simulink library "inp"  (R2021b)
settings: Solver=VariableStepAuto  StartTime=0.0  StopTime=10.0  RelTol=1e-3
undefined symbols (not defined in the file): C_TASK_5MS_S, FALSE, KINP_AcoreReadyToSlp_flg_ovrdflg, KINP_AcoreReadyToSlp_flg_ovrdval, KINP_AllowMovThd_OTA_enum_ovrdflg, KINP_AllowMovThd_OTA_enum_ovrdval, KINP_APSAngleTarget_Deg_ovrdflg, KINP_APSAngleTarget_Deg_ovrdval, KINP_APSDecReq_mps2_ovrdflg, KINP_APSDecReq_mps2_ovrdval, KINP_APSDecReqA_flg_ovrdflg, KINP_APSDecReqA_flg_ovrdval, KINP_APSDFLL_cm_ovrdflg, KINP_APSDFLL_cm_ovrdval, KINP_APSDFLR_cm_ovrdflg, KINP_APSDFLR_cm_ovrdval, KINP_APSDRLL_cm_ovrdflg, KINP_APSDRLL_cm_ovrdval, KINP_APSDRLR_cm_ovrdflg, KINP_APSDRLR_cm_ovrdval, KINP_APSExitCondition_enum_ovrdflg, KINP_APSExitCondition_enum_ovrdval, KINP_APSHWVer_enum_ovrdflg, KINP_APSHWVer_enum_ovrdval, KINP_APSProgressPCT_pct_ovrdflg, KINP_APSProgressPCT_pct_ovrdval, KINP_APSPwrReq_enum_ovrdflg, KINP_APSPwrReq_enum_ovrdval, KINP_APSReq_enum_ovrdflg, KINP_APSReq_enum_ovrdval, KINP_APSRQDisplay_enum_ovrdflg, KINP_APSRQDisplay_enum_ovrdval, KINP_APSRqEPASCtrl_flg_ovrdflg, KINP_APSRqEPASCtrl_flg_ovrdval, KINP_APSShiftPosnReq_enum_ovrdval, KINP_APSShiftPosnReq_enum_ovrflg, KINP_APSSpeedCMD_kph_ovrdval, KINP_APSSpeedCMD_kph_ovrflg, KINP_APSStaSystem_enum_ovrdflg, KINP_APSStaSystem_enum_ovrdval, KINP_APSSWVer_enum_ovrdflg, KINP_APSSWVer_enum_ovrdval, KINP_APSVMCReqA_flg_ovrdval, KINP_APSVMCReqA_flg_ovrflg, KINP_APSVRqEPASCtrl_flg_ovrdflg, KINP_APSVRqEPASCtrl_flg_ovrdval, KINP_AuxBattVolmV_mV_ovrdflg, KINP_AuxBattVolmV_mV_ovrdval, KINP_CAASSta_enum_ovrdflg, KINP_CAASSta_enum_ovrdval, KINP_CAASVMCReqA_flg_ovrdval, KINP_CAASVMCReqA_flg_ovrflg, KINP_CAN1BusOff_flg_ovrdflg, KINP_CAN1BusOff_flg_ovrdval, KINP_CAN2BusOff_flg_ovrdflg, KINP_CAN2BusOff_flg_ovrdval, KINP_CAN3BusOff_flg_ovrdflg, KINP_CAN3BusOff_flg_ovrdval, KINP_CAN4BusOff_flg_ovrdflg, KINP_CAN4BusOff_flg_ovrdval ... (+152)
libraries: FVT_lib x1037, hcu_lib x1
(part 31 of 34)

== system inp/INP/CAN4/SignalCheck/zGW_LINDr2 ==
  BHAL_outputs : Inport
  inp_CanValid_bus : Inport  Port=2
  ACT1ResponseError : FVT_lib/inp/can_signal_template  SystemSampleTime=-1  VariantActivationTime=update diagram  Latency=0  AutoFrameSizeCalculation=off
      link override defval: Value=KINP_ACT1ResponseError_flg_defval
      link override ovrdflg: Value=KINP_ACT1ResponseError_flg_ovrdflg
      link override ovrdval: Value=KINP_ACT1ResponseError_flg_ovrdval
  Terminator_1 : Terminator
  True_VHAL_ACT1ResponseError_flg : Constant  Value=TRUE  OutDataTypeStr=boolean
  slr1_1 : BusSelector  OutputSignals=VINP_CANMsgValidzGWLINDr2_flg
  slr_VHAL_ACT1ResponseError_flg : BusSelector  OutputSignals=VHAL_ACT1ResponseError_flg
  VINP_ACT1ResponseError_flg : Outport
  wires:
  BHAL_outputs/1 -> [BHAL_outputs]
  inp_CanValid_bus/1 -> [inp_CanValid_bus]
  [BHAL_outputs] -> slr_VHAL_ACT1ResponseError_flg/1
  slr_VHAL_ACT1ResponseError_flg/1 -> ACT1ResponseError/1  "<VHAL_ACT1ResponseError_flg>"
  True_VHAL_ACT1ResponseError_flg/1 -> ACT1ResponseError/2
  [inp_CanValid_bus] -> slr1_1/1
  slr1_1/1 -> ACT1ResponseError/3  "<VINP_CANMsgValidzGWLINDr2_flg>"
  ACT1ResponseError/1 -> VINP_ACT1ResponseError_flg/1  "VINP_ACT1ResponseError_flg"
  ACT1ResponseError/2 -> Terminator_1/1

== system inp/INP/CAN4/SignalCheck/zGW_LINFr1 ==
  BHAL_outputs : Inport
  inp_CanValid_bus : Inport  Port=2
  AGSActualPosition : FVT_lib/inp/can_signal_template  SystemSampleTime=-1  VariantActivationTime=update diagram  Latency=0  AutoFrameSizeCalculation=off
      link override defval: Value=KINP_AGSActualPosition_enum_defval
      link override ovrdflg: Value=KINP_AGSActualPosition_enum_ovrdflg
      link override ovrdval: Value=KINP_AGSActualPosition_enum_ovrdval
  FGSIntenRspSta : FVT_lib/inp/can_signal_template  SystemSampleTime=-1  VariantActivationTime=update diagram  Latency=0  AutoFrameSizeCalculation=off
      link override defval: Value=KINP_FGSIntenRspSta_enum_defval
      link override ovrdflg: Value=KINP_FGSIntenRspSta_enum_ovrdflg
      link override ovrdval: Value=KINP_FGSIntenRspSta_enum_ovrdval
  Terminator_1 : Terminator
  Terminator_2 : Terminator
  True_VHAL_AGSActualPosition_enum : Constant  Value=TRUE  OutDataTypeStr=boolean
  True_VHAL_FGSIntenRspSta_enum : Constant  Value=TRUE  OutDataTypeStr=boolean
  slr1_1 : BusSelector  OutputSignals=VINP_CANMsgValidzGWLINFr1_flg
  slr1_2 : BusSelector  OutputSignals=VINP_CANMsgValidzGWLINFr1_flg
  slr_VHAL_AGSActualPosition_enum : BusSelector  OutputSignals=VHAL_AGSActualPosition_enum
  slr_VHAL_FGSIntenRspSta_enum : BusSelector  OutputSignals=VHAL_FGSIntenRspSta_enum
  VINP_AGSActualPosition_enum : Outport
  VINP_FGSIntenRspSta_enum : Outport  Port=2
  wires:
  BHAL_outputs/1 -> [BHAL_outputs]
  inp_CanValid_bus/1 -> [inp_CanValid_bus]
  [BHAL_outputs] -> slr_VHAL_AGSActualPosition_enum/1
  slr_VHAL_AGSActualPosition_enum/1 -> AGSActualPosition/1  "<VHAL_AGSActualPosition_enum>"
  True_VHAL_AGSActualPosition_enum/1 -> AGSActualPosition/2
  [inp_CanValid_bus] -> slr1_1/1
  slr1_1/1 -> AGSActualPosition/3  "<VINP_CANMsgValidzGWLINFr1_flg>"
  AGSActualPosition/1 -> VINP_AGSActualPosition_enum/1  "VINP_AGSActualPosition_enum"
  AGSActualPosition/2 -> Terminator_1/1
  [BHAL_outputs] -> slr_VHAL_FGSIntenRspSta_enum/1
  slr_VHAL_FGSIntenRspSta_enum/1 -> FGSIntenRspSta/1  "<VHAL_FGSIntenRspSta_enum>"
  True_VHAL_FGSIntenRspSta_enum/1 -> FGSIntenRspSta/2
  [inp_CanValid_bus] -> slr1_2/1
  slr1_2/1 -> FGSIntenRspSta/3  "<VINP_CANMsgValidzGWLINFr1_flg>"
  FGSIntenRspSta/1 -> VINP_FGSIntenRspSta_enum/1  "VINP_FGSIntenRspSta_enum"
  FGSIntenRspSta/2 -> Terminator_2/1

== system inp/INP/CAN4/SignalCheck/zGW_LINFr2 ==
  BHAL_outputs : Inport
  inp_CanValid_bus : Inport  Port=2
  EWP1BlockError : FVT_lib/inp/can_signal_template  SystemSampleTime=-1  VariantActivationTime=update diagram  Latency=0  AutoFrameSizeCalculation=off
      link override defval: Value=KINP_EWP1BlockError_enum_defval
      link override ovrdflg: Value=KINP_EWP1BlockError_enum_ovrdflg
      link override ovrdval: Value=KINP_EWP1BlockError_enum_ovrdval
  EWP1OverCurrError : FVT_lib/inp/can_signal_template  SystemSampleTime=-1  VariantActivationTime=update diagram  Latency=0  AutoFrameSizeCalculation=off
      link override defval: Value=KINP_EWP1OverCurrError_enum_defval
      link override ovrdflg: Value=KINP_EWP1OverCurrError_enum_ovrdflg
      link override ovrdval: Value=KINP_EWP1OverCurrError_enum_ovrdval
  EWP2BlockError : FVT_lib/inp/can_signal_template  SystemSampleTime=-1  VariantActivationTime=update diagram  Latency=0  AutoFrameSizeCalculation=off
      link override defval: Value=KINP_EWP2BlockError_enum_defval
      link override ovrdflg: Value=KINP_EWP2BlockError_enum_ovrdflg
      link override ovrdval: Value=KINP_EWP2BlockError_enum_ovrdval
  EWP2OverCurrError : FVT_lib/inp/can_signal_template  SystemSampleTime=-1  VariantActivationTime=update diagram  Latency=0  AutoFrameSizeCalculation=off
      link override defval: Value=KINP_EWP2OverCurrError_enum_defval
      link override ovrdflg: Value=KINP_EWP2OverCurrError_enum_ovrdflg
      link override ovrdval: Value=KINP_EWP2OverCurrError_enum_ovrdval
  EWP3BlockError : FVT_lib/inp/can_signal_template  SystemSampleTime=-1  VariantActivationTime=update diagram  Latency=0  AutoFrameSizeCalculation=off
      link override defval: Value=KINP_EWP3BlockError_enum_defval
      link override ovrdflg: Value=KINP_EWP3BlockError_enum_ovrdflg
      link override ovrdval: Value=KINP_EWP3BlockError_enum_ovrdval
  EWP3OverCurrError : FVT_lib/inp/can_signal_template  SystemSampleTime=-1  VariantActivationTime=update diagram  Latency=0  AutoFrameSizeCalculation=off
      link override defval: Value=KINP_EWP3OverCurrError_enum_defval
      link override ovrdflg: Value=KINP_EWP3OverCurrError_enum_ovrdflg
      link override ovrdval: Value=KINP_EWP3OverCurrError_enum_ovrdval
  Terminator_{1..6} (6 alike) : Terminator
  True_VHAL_EWP1BlockError_enum : Constant  Value=TRUE  OutDataTypeStr=boolean
  True_VHAL_EWP1OverCurrError_enum : Constant  Value=TRUE  OutDataTypeStr=boolean
  True_VHAL_EWP2BlockError_enum : Constant  Value=TRUE  OutDataTypeStr=boolean
  True_VHAL_EWP2OverCurrError_enum : Constant  Value=TRUE  OutDataTypeStr=boolean
  True_VHAL_EWP3BlockError_enum : Constant  Value=TRUE  OutDataTypeStr=boolean
  True_VHAL_EWP3OverCurrError_enum : Constant  Value=TRUE  OutDataTypeStr=boolean
  slr1_{1..6} (6 alike) : BusSelector  OutputSignals=VINP_CANMsgValidzGWLINFr2_flg
  slr_VHAL_EWP1BlockError_enum : BusSelector  OutputSignals=VHAL_EWP1BlockError_enum
  slr_VHAL_EWP1OverCurrError_enum : BusSelector  OutputSignals=VHAL_EWP1OverCurrError_enum
  slr_VHAL_EWP2BlockError_enum : BusSelector  OutputSignals=VHAL_EWP2BlockError_enum
  slr_VHAL_EWP2OverCurrError_enum : BusSelector  OutputSignals=VHAL_EWP2OverCurrError_enum
  slr_VHAL_EWP3BlockError_enum : BusSelector  OutputSignals=VHAL_EWP3BlockError_enum
  slr_VHAL_EWP3OverCurrError_enum : BusSelector  OutputSignals=VHAL_EWP3OverCurrError_enum
  VINP_EWP1BlockError_enum : Outport
  VINP_EWP1OverCurrError_enum : Outport  Port=2
  VINP_EWP2BlockError_enum : Outport  Port=3
  VINP_EWP2OverCurrError_enum : Outport  Port=4
  VINP_EWP3BlockError_enum : Outport  Port=5
  VINP_EWP3OverCurrError_enum : Outport  Port=6
  wires:
  BHAL_outputs/1 -> [BHAL_outputs]
  inp_CanValid_bus/1 -> [inp_CanValid_bus]
  [BHAL_outputs] -> slr_VHAL_EWP1BlockError_enum/1
  slr_VHAL_EWP1BlockError_enum/1 -> EWP1BlockError/1  "<VHAL_EWP1BlockError_enum>"
  True_VHAL_EWP1BlockError_enum/1 -> EWP1BlockError/2
  [inp_CanValid_bus] -> slr1_1/1
  slr1_1/1 -> EWP1BlockError/3  "<VINP_CANMsgValidzGWLINFr2_flg>"
  EWP1BlockError/1 -> VINP_EWP1BlockError_enum/1  "VINP_EWP1BlockError_enum"
  EWP1BlockError/2 -> Terminator_1/1
  [BHAL_outputs] -> slr_VHAL_EWP1OverCurrError_enum/1
  slr_VHAL_EWP1OverCurrError_enum/1 -> EWP1OverCurrError/1  "<VHAL_EWP1OverCurrError_enum>"
  True_VHAL_EWP1OverCurrError_enum/1 -> EWP1OverCurrError/2
  [inp_CanValid_bus] -> slr1_2/1
  slr1_2/1 -> EWP1OverCurrError/3  "<VINP_CANMsgValidzGWLINFr2_flg>"
  EWP1OverCurrError/1 -> VINP_EWP1OverCurrError_enum/1  "VINP_EWP1OverCurrError_enum"
  EWP1OverCurrError/2 -> Terminator_2/1
  [BHAL_outputs] -> slr_VHAL_EWP2BlockError_enum/1
  slr_VHAL_EWP2BlockError_enum/1 -> EWP2BlockError/1  "<VHAL_EWP2BlockError_enum>"
  True_VHAL_EWP2BlockError_enum/1 -> EWP2BlockError/2
  [inp_CanValid_bus] -> slr1_3/1
  slr1_3/1 -> EWP2BlockError/3  "<VINP_CANMsgValidzGWLINFr2_flg>"
  EWP2BlockError/1 -> VINP_EWP2BlockError_enum/1  "VINP_EWP2BlockError_enum"
  EWP2BlockError/2 -> Terminator_3/1
  [BHAL_outputs] -> slr_VHAL_EWP2OverCurrError_enum/1
  slr_VHAL_EWP2OverCurrError_enum/1 -> EWP2OverCurrError/1  "<VHAL_EWP2OverCurrError_enum>"
  True_VHAL_EWP2OverCurrError_enum/1 -> EWP2OverCurrError/2
  [inp_CanValid_bus] -> slr1_4/1
  slr1_4/1 -> EWP2OverCurrError/3  "<VINP_CANMsgValidzGWLINFr2_flg>"
  EWP2OverCurrError/1 -> VINP_EWP2OverCurrError_enum/1  "VINP_EWP2OverCurrError_enum"
  EWP2OverCurrError/2 -> Terminator_4/1
  [BHAL_outputs] -> slr_VHAL_EWP3BlockError_enum/1
  slr_VHAL_EWP3BlockError_enum/1 -> EWP3BlockError/1  "<VHAL_EWP3BlockError_enum>"
  True_VHAL_EWP3BlockError_enum/1 -> EWP3BlockError/2
  [inp_CanValid_bus] -> slr1_5/1
  slr1_5/1 -> EWP3BlockError/3  "<VINP_CANMsgValidzGWLINFr2_flg>"
  EWP3BlockError/1 -> VINP_EWP3BlockError_enum/1  "VINP_EWP3BlockError_enum"
  EWP3BlockError/2 -> Terminator_5/1
  [BHAL_outputs] -> slr_VHAL_EWP3OverCurrError_enum/1
  slr_VHAL_EWP3OverCurrError_enum/1 -> EWP3OverCurrError/1  "<VHAL_EWP3OverCurrError_enum>"
  True_VHAL_EWP3OverCurrError_enum/1 -> EWP3OverCurrError/2
  [inp_CanValid_bus] -> slr1_6/1
  slr1_6/1 -> EWP3OverCurrError/3  "<VINP_CANMsgValidzGWLINFr2_flg>"
  EWP3OverCurrError/1 -> VINP_EWP3OverCurrError_enum/1  "VINP_EWP3OverCurrError_enum"
  EWP3OverCurrError/2 -> Terminator_6/1

== system inp/INP/CAN4/SignalCheck/zGW_SEAT1 ==
  BHAL_outputs : Inport
  inp_CanValid_bus : Inport  Port=2
  DSEATAntiSta : FVT_lib/inp/can_signal_template  SystemSampleTime=-1  VariantActivationTime=update diagram  Latency=0  AutoFrameSizeCalculation=off
      link override defval: Value=KINP_DSEATAntiSta_flg_defval
      link override ovrdflg: Value=KINP_DSEATAntiSta_flg_ovrdflg
      link override ovrdval: Value=KINP_DSEATAntiSta_flg_ovrdval
  DSEATEntryFunSta : FVT_lib/inp/can_signal_template  SystemSampleTime=-1  VariantActivationTime=update diagram  Latency=0  AutoFrameSizeCalculation=off
      link override defval: Value=KINP_DSEATEntryFunSta_flg_defval
      link override ovrdflg: Value=KINP_DSEATEntryFunSta_flg_ovrdflg
      link override ovrdval: Value=KINP_DSEATEntryFunSta_flg_ovrdval
  DSEATErrorSta : FVT_lib/inp/can_signal_template  SystemSampleTime=-1  VariantActivationTime=update diagram  Latency=0  AutoFrameSizeCalculation=off
      link override defval: Value=KINP_DSEATErrorSta_flg_defval
      link override ovrdflg: Value=KINP_DSEATErrorSta_flg_ovrdflg
      link override ovrdval: Value=KINP_DSEATErrorSta_flg_ovrdval
  DSEATHWVer : FVT_lib/inp/can_signal_template  SystemSampleTime=-1  VariantActivationTime=update diagram  Latency=0  AutoFrameSizeCalculation=off
      link override defval: Value=KINP_DSEATHWVer_enum_defval
      link override ovrdflg: Value=KINP_DSEATHWVer_enum_ovrdflg
      link override ovrdval: Value=KINP_DSEATHWVer_enum_ovrdval
  DSEATMode : FVT_lib/inp/can_signal_template  SystemSampleTime=-1  VariantActivationTime=update diagram  Latency=0  AutoFrameSizeCalculation=off
      link override defval: Value=KINP_DSEATMode_enum_defval
      link override ovrdflg: Value=KINP_DSEATMode_enum_ovrdflg
      link override ovrdval: Value=KINP_DSEATMode_enum_ovrdval
  DSEATSWVer : FVT_lib/inp/can_signal_template  SystemSampleTime=-1  VariantActivationTime=update diagram  Latency=0  AutoFrameSizeCalculation=off
      link override defval: Value=KINP_DSEATSWVer_enum_defval
      link override ovrdflg: Value=KINP_DSEATSWVer_enum_ovrdflg
      link override ovrdval: Value=KINP_DSEATSWVer_enum_ovrdval
  DSEATVentSta : FVT_lib/inp/can_signal_template  SystemSampleTime=-1  VariantActivationTime=update diagram  Latency=0  AutoFrameSizeCalculation=off
      link override defval: Value=KINP_DSEATVentSta_enum_defval
      link override ovrdflg: Value=KINP_DSEATVentSta_enum_ovrdflg
      link override ovrdval: Value=KINP_DSEATVentSta_enum_ovrdval
  DSEATheatersta : FVT_lib/inp/can_signal_template  SystemSampleTime=-1  VariantActivationTime=update diagram  Latency=0  AutoFrameSizeCalculation=off
      link override defval: Value=KINP_DSEATheatersta_enum_defval
      link override ovrdflg: Value=KINP_DSEATheatersta_enum_ovrdflg
      link override ovrdval: Value=KINP_DSEATheatersta_enum_ovrdval
  PSEATErrorSta : FVT_lib/inp/can_signal_template  SystemSampleTime=-1  VariantActivationTime=update diagram  Latency=0  AutoFrameSizeCalculation=off
      link override defval: Value=KINP_PSEATErrorSta_flg_defval
      link override ovrdflg: Value=KINP_PSEATErrorSta_flg_ovrdflg
      link override ovrdval: Value=KINP_PSEATErrorSta_flg_ovrdval
  PSEATHWVer : FVT_lib/inp/can_signal_template  SystemSampleTime=-1  VariantActivationTime=update diagram  Latency=0  AutoFrameSizeCalculation=off
      link override defval: Value=KINP_PSEATHWVer_enum_defval
      link override ovrdflg: Value=KINP_PSEATHWVer_enum_ovrdflg
      link override ovrdval: Value=KINP_PSEATHWVer_enum_ovrdval
  PSEATMode : FVT_lib/inp/can_signal_template  SystemSampleTime=-1  VariantActivationTime=update diagram  Latency=0  AutoFrameSizeCalculation=off
      link override defval: Value=KINP_PSEATMode_enum_defval
      link override ovrdflg: Value=KINP_PSEATMode_enum_ovrdflg
      link override ovrdval: Value=KINP_PSEATMode_enum_ovrdval
  PSEATSWVer : FVT_lib/inp/can_signal_template  SystemSampleTime=-1  VariantActivationTime=update diagram  Latency=0  AutoFrameSizeCalculation=off
      link override defval: Value=KINP_PSEATSWVer_enum_defval
      link override ovrdflg: Value=KINP_PSEATSWVer_enum_ovrdflg
      link override ovrdval: Value=KINP_PSEATSWVer_enum_ovrdval
  PSEATVentSta : FVT_lib/inp/can_signal_template  SystemSampleTime=-1  VariantActivationTime=update diagram  Latency=0  AutoFrameSizeCalculation=off
      link override defval: Value=KINP_PSEATVentSta_enum_defval
      link override ovrdflg: Value=KINP_PSEATVentSta_enum_ovrdflg
      link override ovrdval: Value=KINP_PSEATVentSta_enum_ovrdval
  PSEATheatersta : FVT_lib/inp/can_signal_template  SystemSampleTime=-1  VariantActivationTime=update diagram  Latency=0  AutoFrameSizeCalculation=off
      link override defval: Value=KINP_PSEATheatersta_enum_defval
      link override ovrdflg: Value=KINP_PSEATheatersta_enum_ovrdflg
      link override ovrdval: Value=KINP_PSEATheatersta_enum_ovrdval
  Terminator_{1..14} (14 alike) : Terminator
  True_VHAL_DSEATAntiSta_flg : Constant  Value=TRUE  OutDataTypeStr=boolean
  True_VHAL_DSEATEntryFunSta_flg : Constant  Value=TRUE  OutDataTypeStr=boolean
  True_VHAL_DSEATErrorSta_flg : Constant  Value=TRUE  OutDataTypeStr=boolean
  True_VHAL_DSEATHWVer_enum : Constant  Value=TRUE  OutDataTypeStr=boolean
  True_VHAL_DSEATMode_enum : Constant  Value=TRUE  OutDataTypeStr=boolean
  True_VHAL_DSEATSWVer_enum : Constant  Value=TRUE  OutDataTypeStr=boolean
  True_VHAL_DSEATVentSta_enum : Constant  Value=TRUE  OutDataTypeStr=boolean
  True_VHAL_DSEATheatersta_enum : Constant  Value=TRUE  OutDataTypeStr=boolean
  True_VHAL_PSEATErrorSta_flg : Constant  Value=TRUE  OutDataTypeStr=boolean
  True_VHAL_PSEATHWVer_enum : Constant  Value=TRUE  OutDataTypeStr=boolean
  True_VHAL_PSEATMode_enum : Constant  Value=TRUE  OutDataTypeStr=boolean
  True_VHAL_PSEATSWVer_enum : Constant  Value=TRUE  OutDataTypeStr=boolean
  True_VHAL_PSEATVentSta_enum : Constant  Value=TRUE  OutDataTypeStr=boolean
  True_VHAL_PSEATheatersta_enum : Constant  Value=TRUE  OutDataTypeStr=boolean
  slr1_{1..14} (14 alike) : BusSelector  OutputSignals=VINP_CANMsgValidzGWSEAT1_flg
  slr_VHAL_DSEATAntiSta_flg : BusSelector  OutputSignals=VHAL_DSEATAntiSta_flg
  slr_VHAL_DSEATEntryFunSta_flg : BusSelector  OutputSignals=VHAL_DSEATEntryFunSta_flg
  slr_VHAL_DSEATErrorSta_flg : BusSelector  OutputSignals=VHAL_DSEATErrorSta_flg
  slr_VHAL_DSEATHWVer_enum : BusSelector  OutputSignals=VHAL_DSEATHWVer_enum
  slr_VHAL_DSEATMode_enum : BusSelector  OutputSignals=VHAL_DSEATMode_enum
  slr_VHAL_DSEATSWVer_enum : BusSelector  OutputSignals=VHAL_DSEATSWVer_enum
  slr_VHAL_DSEATVentSta_enum : BusSelector  OutputSignals=VHAL_DSEATVentSta_enum
  slr_VHAL_DSEATheatersta_enum : BusSelector  OutputSignals=VHAL_DSEATheatersta_enum
  slr_VHAL_PSEATErrorSta_flg : BusSelector  OutputSignals=VHAL_PSEATErrorSta_flg
  slr_VHAL_PSEATHWVer_enum : BusSelector  OutputSignals=VHAL_PSEATHWVer_enum
  slr_VHAL_PSEATMode_enum : BusSelector  OutputSignals=VHAL_PSEATMode_enum
  slr_VHAL_PSEATSWVer_enum : BusSelector  OutputSignals=VHAL_PSEATSWVer_enum
  slr_VHAL_PSEATVentSta_enum : BusSelector  OutputSignals=VHAL_PSEATVentSta_enum
  slr_VHAL_PSEATheatersta_enum : BusSelector  OutputSignals=VHAL_PSEATheatersta_enum
  VINP_DSEATAntiSta_flg : Outport
  VINP_DSEATEntryFunSta_flg : Outport  Port=2
  VINP_DSEATErrorSta_flg : Outport  Port=3
  VINP_DSEATHWVer_enum : Outport  Port=4
  VINP_DSEATMode_enum : Outport  Port=5
  VINP_DSEATSWVer_enum : Outport  Port=6
  VINP_DSEATVentSta_enum : Outport  Port=7
  VINP_DSEATheatersta_enum : Outport  Port=8
  VINP_PSEATErrorSta_flg : Outport  Port=9
  VINP_PSEATHWVer_enum : Outport  Port=10
  VINP_PSEATMode_enum : Outport  Port=11
  VINP_PSEATSWVer_enum : Outport  Port=12
  VINP_PSEATVentSta_enum : Outport  Port=13
  VINP_PSEATheatersta_enum : Outport  Port=14
  wires:
  BHAL_outputs/1 -> [BHAL_outputs]
  inp_CanValid_bus/1 -> [inp_CanValid_bus]
  [BHAL_outputs] -> slr_VHAL_DSEATAntiSta_flg/1
  slr_VHAL_DSEATAntiSta_flg/1 -> DSEATAntiSta/1  "<VHAL_DSEATAntiSta_flg>"
  True_VHAL_DSEATAntiSta_flg/1 -> DSEATAntiSta/2
  [inp_CanValid_bus] -> slr1_1/1
  slr1_1/1 -> DSEATAntiSta/3  "<VINP_CANMsgValidzGWSEAT1_flg>"
  DSEATAntiSta/1 -> VINP_DSEATAntiSta_flg/1  "VINP_DSEATAntiSta_flg"
  DSEATAntiSta/2 -> Terminator_1/1
  [BHAL_outputs] -> slr_VHAL_DSEATEntryFunSta_flg/1
  slr_VHAL_DSEATEntryFunSta_flg/1 -> DSEATEntryFunSta/1  "<VHAL_DSEATEntryFunSta_flg>"
  True_VHAL_DSEATEntryFunSta_flg/1 -> DSEATEntryFunSta/2
  [inp_CanValid_bus] -> slr1_2/1
  slr1_2/1 -> DSEATEntryFunSta/3  "<VINP_CANMsgValidzGWSEAT1_flg>"
  DSEATEntryFunSta/1 -> VINP_DSEATEntryFunSta_flg/1  "VINP_DSEATEntryFunSta_flg"
  DSEATEntryFunSta/2 -> Terminator_2/1
  [BHAL_outputs] -> slr_VHAL_DSEATErrorSta_flg/1
  slr_VHAL_DSEATErrorSta_flg/1 -> DSEATErrorSta/1  "<VHAL_DSEATErrorSta_flg>"
  True_VHAL_DSEATErrorSta_flg/1 -> DSEATErrorSta/2
  [inp_CanValid_bus] -> slr1_3/1
  slr1_3/1 -> DSEATErrorSta/3  "<VINP_CANMsgValidzGWSEAT1_flg>"
  DSEATErrorSta/1 -> VINP_DSEATErrorSta_flg/1  "VINP_DSEATErrorSta_flg"
  DSEATErrorSta/2 -> Terminator_3/1
  [BHAL_outputs] -> slr_VHAL_DSEATHWVer_enum/1
  slr_VHAL_DSEATHWVer_enum/1 -> DSEATHWVer/1  "<VHAL_DSEATHWVer_enum>"
  True_VHAL_DSEATHWVer_enum/1 -> DSEATHWVer/2
  [inp_CanValid_bus] -> slr1_4/1
  slr1_4/1 -> DSEATHWVer/3  "<VINP_CANMsgValidzGWSEAT1_flg>"
  DSEATHWVer/1 -> VINP_DSEATHWVer_enum/1  "VINP_DSEATHWVer_enum"
  DSEATHWVer/2 -> Terminator_4/1
  [BHAL_outputs] -> slr_VHAL_DSEATMode_enum/1
  slr_VHAL_DSEATMode_enum/1 -> DSEATMode/1  "<VHAL_DSEATMode_enum>"
  True_VHAL_DSEATMode_enum/1 -> DSEATMode/2
  [inp_CanValid_bus] -> slr1_5/1
  slr1_5/1 -> DSEATMode/3  "<VINP_CANMsgValidzGWSEAT1_flg>"
  DSEATMode/1 -> VINP_DSEATMode_enum/1  "VINP_DSEATMode_enum"
  DSEATMode/2 -> Terminator_5/1
  [BHAL_outputs] -> slr_VHAL_DSEATSWVer_enum/1
  slr_VHAL_DSEATSWVer_enum/1 -> DSEATSWVer/1  "<VHAL_DSEATSWVer_enum>"
  True_VHAL_DSEATSWVer_enum/1 -> DSEATSWVer/2
  [inp_CanValid_bus] -> slr1_6/1
  slr1_6/1 -> DSEATSWVer/3  "<VINP_CANMsgValidzGWSEAT1_flg>"
  DSEATSWVer/1 -> VINP_DSEATSWVer_enum/1  "VINP_DSEATSWVer_enum"
  DSEATSWVer/2 -> Terminator_6/1
  [BHAL_outputs] -> slr_VHAL_DSEATVentSta_enum/1
  slr_VHAL_DSEATVentSta_enum/1 -> DSEATVentSta/1  "<VHAL_DSEATVentSta_enum>"
  True_VHAL_DSEATVentSta_enum/1 -> DSEATVentSta/2
  [inp_CanValid_bus] -> slr1_7/1
  slr1_7/1 -> DSEATVentSta/3  "<VINP_CANMsgValidzGWSEAT1_flg>"
  DSEATVentSta/1 -> VINP_DSEATVentSta_enum/1  "VINP_DSEATVentSta_enum"
  DSEATVentSta/2 -> Terminator_7/1
  [BHAL_outputs] -> slr_VHAL_DSEATheatersta_enum/1
  slr_VHAL_DSEATheatersta_enum/1 -> DSEATheatersta/1  "<VHAL_DSEATheatersta_enum>"
  True_VHAL_DSEATheatersta_enum/1 -> DSEATheatersta/2
  [inp_CanValid_bus] -> slr1_8/1
  slr1_8/1 -> DSEATheatersta/3  "<VINP_CANMsgValidzGWSEAT1_flg>"
  DSEATheatersta/1 -> VINP_DSEATheatersta_enum/1  "VINP_DSEATheatersta_enum"
  DSEATheatersta/2 -> Terminator_8/1
  [BHAL_outputs] -> slr_VHAL_PSEATErrorSta_flg/1
  slr_VHAL_PSEATErrorSta_flg/1 -> PSEATErrorSta/1  "<VHAL_PSEATErrorSta_flg>"
  True_VHAL_PSEATErrorSta_flg/1 -> PSEATErrorSta/2
  [inp_CanValid_bus] -> slr1_9/1
  slr1_9/1 -> PSEATErrorSta/3  "<VINP_CANMsgValidzGWSEAT1_flg>"
  PSEATErrorSta/1 -> VINP_PSEATErrorSta_flg/1  "VINP_PSEATErrorSta_flg"
  PSEATErrorSta/2 -> Terminator_9/1
  [BHAL_outputs] -> slr_VHAL_PSEATHWVer_enum/1
  slr_VHAL_PSEATHWVer_enum/1 -> PSEATHWVer/1  "<VHAL_PSEATHWVer_enum>"
  True_VHAL_PSEATHWVer_enum/1 -> PSEATHWVer/2
  [inp_CanValid_bus] -> slr1_10/1
  slr1_10/1 -> PSEATHWVer/3  "<VINP_CANMsgValidzGWSEAT1_flg>"
  PSEATHWVer/1 -> VINP_PSEATHWVer_enum/1  "VINP_PSEATHWVer_enum"
  PSEATHWVer/2 -> Terminator_10/1
  [BHAL_outputs] -> slr_VHAL_PSEATMode_enum/1
  slr_VHAL_PSEATMode_enum/1 -> PSEATMode/1  "<VHAL_PSEATMode_enum>"
  True_VHAL_PSEATMode_enum/1 -> PSEATMode/2
  [inp_CanValid_bus] -> slr1_11/1
  slr1_11/1 -> PSEATMode/3  "<VINP_CANMsgValidzGWSEAT1_flg>"
  PSEATMode/1 -> VINP_PSEATMode_enum/1  "VINP_PSEATMode_enum"
  PSEATMode/2 -> Terminator_11/1
  [BHAL_outputs] -> slr_VHAL_PSEATSWVer_enum/1
  slr_VHAL_PSEATSWVer_enum/1 -> PSEATSWVer/1  "<VHAL_PSEATSWVer_enum>"
  True_VHAL_PSEATSWVer_enum/1 -> PSEATSWVer/2
  [inp_CanValid_bus] -> slr1_12/1
  slr1_12/1 -> PSEATSWVer/3  "<VINP_CANMsgValidzGWSEAT1_flg>"
  PSEATSWVer/1 -> VINP_PSEATSWVer_enum/1  "VINP_PSEATSWVer_enum"
  PSEATSWVer/2 -> Terminator_12/1
  [BHAL_outputs] -> slr_VHAL_PSEATVentSta_enum/1
  slr_VHAL_PSEATVentSta_enum/1 -> PSEATVentSta/1  "<VHAL_PSEATVentSta_enum>"
  True_VHAL_PSEATVentSta_enum/1 -> PSEATVentSta/2
  [inp_CanValid_bus] -> slr1_13/1
  slr1_13/1 -> PSEATVentSta/3  "<VINP_CANMsgValidzGWSEAT1_flg>"
  PSEATVentSta/1 -> VINP_PSEATVentSta_enum/1  "VINP_PSEATVentSta_enum"
  PSEATVentSta/2 -> Terminator_13/1
  [BHAL_outputs] -> slr_VHAL_PSEATheatersta_enum/1
  slr_VHAL_PSEATheatersta_enum/1 -> PSEATheatersta/1  "<VHAL_PSEATheatersta_enum>"
  True_VHAL_PSEATheatersta_enum/1 -> PSEATheatersta/2
  [inp_CanValid_bus] -> slr1_14/1
  slr1_14/1 -> PSEATheatersta/3  "<VINP_CANMsgValidzGWSEAT1_flg>"
  PSEATheatersta/1 -> VINP_PSEATheatersta_enum/1  "VINP_PSEATheatersta_enum"
  PSEATheatersta/2 -> Terminator_14/1

== system inp/INP/CAN5/SignalCheck/TBOX1 ==
  BHAL_outputs : Inport
  inp_CanValid_bus : Inport  Port=2
  CbnPreACEnaReq : FVT_lib/inp/can_signal_template  SystemSampleTime=-1  VariantActivationTime=update diagram  Latency=0  AutoFrameSizeCalculation=off
      link override defval: Value=KINP_CbnPreACEnaReq_enum_defval
      link override ovrdflg: Value=KINP_CbnPreACEnaReq_enum_ovrdflg
      link override ovrdval: Value=KINP_CbnPreACEnaReq_enum_ovrdval
  PowerOffTSet : FVT_lib/inp/can_signal_template  SystemSampleTime=-1  VariantActivationTime=update diagram  Latency=0  AutoFrameSizeCalculation=off
      link override defval: Value=KINP_PowerOffTSet_cnt_defval
      link override ovrdflg: Value=KINP_PowerOffTSet_cnt_ovrdflg
      link override ovrdval: Value=KINP_PowerOffTSet_cnt_ovrdval
  ReDoorLock : FVT_lib/inp/can_signal_template  SystemSampleTime=-1  VariantActivationTime=update diagram  Latency=0  AutoFrameSizeCalculation=off
      link override defval: Value=KINP_ReDoorLock_enum_defval
      link override ovrdflg: Value=KINP_ReDoorLock_enum_ovrdflg
      link override ovrdval: Value=KINP_ReDoorLock_enum_ovrdval
  ReOutsideMirror : FVT_lib/inp/can_signal_template  SystemSampleTime=-1  VariantActivationTime=update diagram  Latency=0  AutoFrameSizeCalculation=off
      link override defval: Value=KINP_ReOutsideMirror_enum_defval
      link override ovrdflg: Value=KINP_ReOutsideMirror_enum_ovrdflg
      link override ovrdval: Value=KINP_ReOutsideMirror_enum_ovrdval
  RePwrReqTbox : FVT_lib/inp/can_signal_template  SystemSampleTime=-1  VariantActivationTime=update diagram  Latency=0  AutoFrameSizeCalculation=off
      link override defval: Value=KINP_RePwrReqTbox_enum_defval
      link override ovrdflg: Value=KINP_RePwrReqTbox_enum_ovrdflg
      link override ovrdval: Value=KINP_RePwrReqTbox_enum_ovrdval
  ReRadio : FVT_lib/inp/can_signal_template  SystemSampleTime=-1  VariantActivationTime=update diagram  Latency=0  AutoFrameSizeCalculation=off
      link override defval: Value=KINP_ReRadio_flg_defval
      link override ovrdflg: Value=KINP_ReRadio_flg_ovrdflg
      link override ovrdval: Value=KINP_ReRadio_flg_ovrdval
  RemoteACTemp : FVT_lib/inp/can_signal_template  SystemSampleTime=-1  VariantActivationTime=update diagram  Latency=0  AutoFrameSizeCalculation=off
      link override defval: Value=KINP_RemoteACTemp_C_defval
      link override ovrdflg: Value=KINP_RemoteACTemp_C_ovrdflg
      link override ovrdval: Value=KINP_RemoteACTemp_C_ovrdval
  RemoteAutoReq : FVT_lib/inp/can_signal_template  SystemSampleTime=-1  VariantActivationTime=update diagram  Latency=0  AutoFrameSizeCalculation=off
      link override defval: Value=KINP_RemoteAutoReq_flg_defval
      link override ovrdflg: Value=KINP_RemoteAutoReq_flg_ovrdflg
      link override ovrdval: Value=KINP_RemoteAutoReq_flg_ovrdval
  TBOXNETSIGSTR : FVT_lib/inp/can_signal_template  SystemSampleTime=-1  VariantActivationTime=update diagram  Latency=0  AutoFrameSizeCalculation=off
      link override defval: Value=KINP_TBOXNETSIGSTR_enum_defval
      link override ovrdflg: Value=KINP_TBOXNETSIGSTR_enum_ovrdflg
      link override ovrdval: Value=KINP_TBOXNETSIGSTR_enum_ovrdval
  TBOXRemotePW : FVT_lib/inp/can_signal_template  SystemSampleTime=-1  VariantActivationTime=update diagram  Latency=0  AutoFrameSizeCalculation=off
      link override defval: Value=KINP_TBOXRemotePW_enum_defval
      link override ovrdflg: Value=KINP_TBOXRemotePW_enum_ovrdflg
      link override ovrdval: Value=KINP_TBOXRemotePW_enum_ovrdval
  TBOXTESTSTATUS : FVT_lib/inp/can_signal_template  SystemSampleTime=-1  VariantActivationTime=update diagram  Latency=0  AutoFrameSizeCalculation=off
      link override defval: Value=KINP_TBOXTESTSTATUS_enum_defval
      link override ovrdflg: Value=KINP_TBOXTESTSTATUS_enum_ovrdflg
      link override ovrdval: Value=KINP_TBOXTESTSTATUS_enum_ovrdval
  Terminator_{1..11} (11 alike) : Terminator
  True_VHAL_CbnPreACEnaReq_enum : Constant  Value=TRUE  OutDataTypeStr=boolean
  True_VHAL_PowerOffTSet_cnt : Constant  Value=TRUE  OutDataTypeStr=boolean
  True_VHAL_ReDoorLock_enum : Constant  Value=TRUE  OutDataTypeStr=boolean
  True_VHAL_ReOutsideMirror_enum : Constant  Value=TRUE  OutDataTypeStr=boolean
  True_VHAL_RePwrReqTbox_enum : Constant  Value=TRUE  OutDataTypeStr=boolean
  True_VHAL_ReRadio_flg : Constant  Value=TRUE  OutDataTypeStr=boolean
  True_VHAL_RemoteACTemp_C : Constant  Value=TRUE  OutDataTypeStr=boolean
  True_VHAL_RemoteAutoReq_flg : Constant  Value=TRUE  OutDataTypeStr=boolean
  True_VHAL_TBOXNETSIGSTR_enum : Constant  Value=TRUE  OutDataTypeStr=boolean
  True_VHAL_TBOXRemotePW_enum : Constant  Value=TRUE  OutDataTypeStr=boolean
  True_VHAL_TBOXTESTSTATUS_enum : Constant  Value=TRUE  OutDataTypeStr=boolean
  slr1_{1..11} (11 alike) : BusSelector  OutputSignals=VINP_CANMsgValidTBOX1_flg
  slr_VHAL_CbnPreACEnaReq_enum : BusSelector  OutputSignals=VHAL_CbnPreACEnaReq_enum
  slr_VHAL_PowerOffTSet_cnt : BusSelector  OutputSignals=VHAL_PowerOffTSet_cnt
  slr_VHAL_ReDoorLock_enum : BusSelector  OutputSignals=VHAL_ReDoorLock_enum
  slr_VHAL_ReOutsideMirror_enum : BusSelector  OutputSignals=VHAL_ReOutsideMirror_enum
  slr_VHAL_RePwrReqTbox_enum : BusSelector  OutputSignals=VHAL_RePwrReqTbox_enum
  slr_VHAL_ReRadio_flg : BusSelector  OutputSignals=VHAL_ReRadio_flg
  slr_VHAL_RemoteACTemp_C : BusSelector  OutputSignals=VHAL_RemoteACTemp_C
  slr_VHAL_RemoteAutoReq_flg : BusSelector  OutputSignals=VHAL_RemoteAutoReq_flg
  slr_VHAL_TBOXNETSIGSTR_enum : BusSelector  OutputSignals=VHAL_TBOXNETSIGSTR_enum
  slr_VHAL_TBOXRemotePW_enum : BusSelector  OutputSignals=VHAL_TBOXRemotePW_enum
  slr_VHAL_TBOXTESTSTATUS_enum : BusSelector  OutputSignals=VHAL_TBOXTESTSTATUS_enum
  VINP_CbnPreACEnaReq_enum : Outport
  VINP_PowerOffTSet_cnt : Outport  Port=2
  VINP_ReOutsideMirror_enum : Outport  Port=3
  VINP_ReDoorLock_enum : Outport  Port=4
  VINP_RePwrReqTbox_enum : Outport  Port=5
  VINP_ReRadio_flg : Outport  Port=6
  VINP_RemoteACTemp_C : Outport  Port=7
  VINP_RemoteAutoReq_flg : Outport  Port=8
  VINP_TBOXNETSIGSTR_enum : Outport  Port=9
  VINP_TBOXRemotePW_enum : Outport  Port=10
  VINP_TBOXTESTSTATUS_enum : Outport  Port=11
  wires:
  BHAL_outputs/1 -> [BHAL_outputs]
  inp_CanValid_bus/1 -> [inp_CanValid_bus]
  [BHAL_outputs] -> slr_VHAL_CbnPreACEnaReq_enum/1
  slr_VHAL_CbnPreACEnaReq_enum/1 -> CbnPreACEnaReq/1  "<VHAL_CbnPreACEnaReq_enum>"
  True_VHAL_CbnPreACEnaReq_enum/1 -> CbnPreACEnaReq/2
  [inp_CanValid_bus] -> slr1_1/1
  slr1_1/1 -> CbnPreACEnaReq/3  "<VINP_CANMsgValidTBOX1_flg>"
  CbnPreACEnaReq/1 -> VINP_CbnPreACEnaReq_enum/1  "VINP_CbnPreACEnaReq_enum"
  CbnPreACEnaReq/2 -> Terminator_1/1
  [BHAL_outputs] -> slr_VHAL_PowerOffTSet_cnt/1
  slr_VHAL_PowerOffTSet_cnt/1 -> PowerOffTSet/1  "<VHAL_PowerOffTSet_cnt>"
  True_VHAL_PowerOffTSet_cnt/1 -> PowerOffTSet/2
  [inp_CanValid_bus] -> slr1_2/1
  slr1_2/1 -> PowerOffTSet/3  "<VINP_CANMsgValidTBOX1_flg>"
  PowerOffTSet/1 -> VINP_PowerOffTSet_cnt/1  "VINP_PowerOffTSet_cnt"
  PowerOffTSet/2 -> Terminator_2/1
  [BHAL_outputs] -> slr_VHAL_ReOutsideMirror_enum/1
  slr_VHAL_ReOutsideMirror_enum/1 -> ReOutsideMirror/1  "<VHAL_ReOutsideMirror_enum>"
  True_VHAL_ReOutsideMirror_enum/1 -> ReOutsideMirror/2
  [inp_CanValid_bus] -> slr1_3/1
  slr1_3/1 -> ReOutsideMirror/3  "<VINP_CANMsgValidTBOX1_flg>"
  ReOutsideMirror/1 -> VINP_ReOutsideMirror_enum/1  "VINP_ReOutsideMirror_enum"
  ReOutsideMirror/2 -> Terminator_3/1
  [BHAL_outputs] -> slr_VHAL_ReDoorLock_enum/1
  slr_VHAL_ReDoorLock_enum/1 -> ReDoorLock/1  "<VHAL_ReDoorLock_enum>"
  True_VHAL_ReDoorLock_enum/1 -> ReDoorLock/2
  [inp_CanValid_bus] -> slr1_4/1
  slr1_4/1 -> ReDoorLock/3  "<VINP_CANMsgValidTBOX1_flg>"
  ReDoorLock/1 -> VINP_ReDoorLock_enum/1  "VINP_ReDoorLock_enum"
  ReDoorLock/2 -> Terminator_4/1
  [BHAL_outputs] -> slr_VHAL_RePwrReqTbox_enum/1
  slr_VHAL_RePwrReqTbox_enum/1 -> RePwrReqTbox/1  "<VHAL_RePwrReqTbox_enum>"
  True_VHAL_RePwrReqTbox_enum/1 -> RePwrReqTbox/2
  [inp_CanValid_bus] -> slr1_5/1
  slr1_5/1 -> RePwrReqTbox/3  "<VINP_CANMsgValidTBOX1_flg>"
  RePwrReqTbox/1 -> VINP_RePwrReqTbox_enum/1  "VINP_RePwrReqTbox_enum"
  RePwrReqTbox/2 -> Terminator_5/1
  [BHAL_outputs] -> slr_VHAL_ReRadio_flg/1
  slr_VHAL_ReRadio_flg/1 -> ReRadio/1  "<VHAL_ReRadio_flg>"
  True_VHAL_ReRadio_flg/1 -> ReRadio/2
  [inp_CanValid_bus] -> slr1_6/1
  slr1_6/1 -> ReRadio/3  "<VINP_CANMsgValidTBOX1_flg>"
  ReRadio/1 -> VINP_ReRadio_flg/1  "VINP_ReRadio_flg"
  ReRadio/2 -> Terminator_6/1
  [BHAL_outputs] -> slr_VHAL_RemoteACTemp_C/1
  slr_VHAL_RemoteACTemp_C/1 -> RemoteACTemp/1  "<VHAL_RemoteACTemp_C>"
  True_VHAL_RemoteACTemp_C/1 -> RemoteACTemp/2
  [inp_CanValid_bus] -> slr1_7/1
  slr1_7/1 -> RemoteACTemp/3  "<VINP_CANMsgValidTBOX1_flg>"
  RemoteACTemp/1 -> VINP_RemoteACTemp_C/1  "VINP_RemoteACTemp_C"
  RemoteACTemp/2 -> Terminator_7/1
  [BHAL_outputs] -> slr_VHAL_RemoteAutoReq_flg/1
  slr_VHAL_RemoteAutoReq_flg/1 -> RemoteAutoReq/1  "<VHAL_RemoteAutoReq_flg>"
  True_VHAL_RemoteAutoReq_flg/1 -> RemoteAutoReq/2
  [inp_CanValid_bus] -> slr1_8/1
  slr1_8/1 -> RemoteAutoReq/3  "<VINP_CANMsgValidTBOX1_flg>"
  RemoteAutoReq/1 -> VINP_RemoteAutoReq_flg/1  "VINP_RemoteAutoReq_flg"
  RemoteAutoReq/2 -> Terminator_8/1
  [BHAL_outputs] -> slr_VHAL_TBOXNETSIGSTR_enum/1
  slr_VHAL_TBOXNETSIGSTR_enum/1 -> TBOXNETSIGSTR/1  "<VHAL_TBOXNETSIGSTR_enum>"
  True_VHAL_TBOXNETSIGSTR_enum/1 -> TBOXNETSIGSTR/2
  [inp_CanValid_bus] -> slr1_9/1
  slr1_9/1 -> TBOXNETSIGSTR/3  "<VINP_CANMsgValidTBOX1_flg>"
  TBOXNETSIGSTR/1 -> VINP_TBOXNETSIGSTR_enum/1  "VINP_TBOXNETSIGSTR_enum"
  TBOXNETSIGSTR/2 -> Terminator_9/1
  [BHAL_outputs] -> slr_VHAL_TBOXRemotePW_enum/1
  slr_VHAL_TBOXRemotePW_enum/1 -> TBOXRemotePW/1  "<VHAL_TBOXRemotePW_enum>"
  True_VHAL_TBOXRemotePW_enum/1 -> TBOXRemotePW/2
  [inp_CanValid_bus] -> slr1_10/1
  slr1_10/1 -> TBOXRemotePW/3  "<VINP_CANMsgValidTBOX1_flg>"
  TBOXRemotePW/1 -> VINP_TBOXRemotePW_enum/1  "VINP_TBOXRemotePW_enum"
  TBOXRemotePW/2 -> Terminator_10/1
  [BHAL_outputs] -> slr_VHAL_TBOXTESTSTATUS_enum/1
  slr_VHAL_TBOXTESTSTATUS_enum/1 -> TBOXTESTSTATUS/1  "<VHAL_TBOXTESTSTATUS_enum>"
  True_VHAL_TBOXTESTSTATUS_enum/1 -> TBOXTESTSTATUS/2
  [inp_CanValid_bus] -> slr1_11/1
  slr1_11/1 -> TBOXTESTSTATUS/3  "<VINP_CANMsgValidTBOX1_flg>"
  TBOXTESTSTATUS/1 -> VINP_TBOXTESTSTATUS_enum/1  "VINP_TBOXTESTSTATUS_enum"
  TBOXTESTSTATUS/2 -> Terminator_11/1

== system inp/INP/CAN5/SignalCheck/TBOX2 ==
  BHAL_outputs : Inport
  inp_CanValid_bus : Inport  Port=2
  Terminator_{1..6} (6 alike) : Terminator
  TimeSyncFromBSDay : FVT_lib/inp/can_signal_template  SystemSampleTime=-1  VariantActivationTime=update diagram  Latency=0  AutoFrameSizeCalculation=off
      link override defval: Value=KINP_TimeSyncFromBSDay_DAY_defval
      link override ovrdflg: Value=KINP_TimeSyncFromBSDay_DAY_ovrdflg
      link override ovrdval: Value=KINP_TimeSyncFromBSDay_DAY_ovrdval
  TimeSyncFromBSHour : FVT_lib/inp/can_signal_template  SystemSampleTime=-1  VariantActivationTime=update diagram  Latency=0  AutoFrameSizeCalculation=off
      link override defval: Value=KINP_TimeSyncFromBSHour_hr_defval
      link override ovrdflg: Value=KINP_TimeSyncFromBSHour_hr_ovrdflg
      link override ovrdval: Value=KINP_TimeSyncFromBSHour_hr_ovrdval
  TimeSyncFromBSMinute : FVT_lib/inp/can_signal_template  SystemSampleTime=-1  VariantActivationTime=update diagram  Latency=0  AutoFrameSizeCalculation=off
      link override defval: Value=KINP_TimeSyncFromBSMinute_min_defval
      link override ovrdflg: Value=KINP_TimeSyncFromBSMinute_min_ovrdflg
      link override ovrdval: Value=KINP_TimeSyncFromBSMinute_min_ovrdval
  TimeSyncFromBSMonth : FVT_lib/inp/can_signal_template  SystemSampleTime=-1  VariantActivationTime=update diagram  Latency=0  AutoFrameSizeCalculation=off
      link override defval: Value=KINP_TimeSyncFromBSMonth_MONTH_defval
      link override ovrdflg: Value=KINP_TimeSyncFromBSMonth_MONTH_ovrdflg
      link override ovrdval: Value=KINP_TimeSyncFromBSMonth_MONTH_ovrdval
  TimeSyncFromBSSecond : FVT_lib/inp/can_signal_template  SystemSampleTime=-1  VariantActivationTime=update diagram  Latency=0  AutoFrameSizeCalculation=off
      link override defval: Value=KINP_TimeSyncFromBSSecond_s_defval
      link override ovrdflg: Value=KINP_TimeSyncFromBSSecond_s_ovrdflg
      link override ovrdval: Value=KINP_TimeSyncFromBSSecond_s_ovrdval
  TimeSyncFromBSYear : FVT_lib/inp/can_signal_template  SystemSampleTime=-1  VariantActivationTime=update diagram  Latency=0  AutoFrameSizeCalculation=off
      link override defval: Value=KINP_TimeSyncFromBSYear_YEAR_defval
      link override ovrdflg: Value=KINP_TimeSyncFromBSYear_YEAR_ovrdflg
      link override ovrdval: Value=KINP_TimeSyncFromBSYear_YEAR_ovrdval
  True_VHAL_TimeSyncFromBSDay_DAY : Constant  Value=TRUE  OutDataTypeStr=boolean
  True_VHAL_TimeSyncFromBSHour_hr : Constant  Value=TRUE  OutDataTypeStr=boolean
  True_VHAL_TimeSyncFromBSMinute_min : Constant  Value=TRUE  OutDataTypeStr=boolean
  True_VHAL_TimeSyncFromBSMonth_MONTH : Constant  Value=TRUE  OutDataTypeStr=boolean
  True_VHAL_TimeSyncFromBSSecond_s : Constant  Value=TRUE  OutDataTypeStr=boolean
  True_VHAL_TimeSyncFromBSYear_YEAR : Constant  Value=TRUE  OutDataTypeStr=boolean
  slr1_{1..6} (6 alike) : BusSelector  OutputSignals=VINP_CANMsgValidTBOX2_flg
  slr_VHAL_TimeSyncFromBSDay_DAY : BusSelector  OutputSignals=VHAL_TimeSyncFromBSDay_DAY
  slr_VHAL_TimeSyncFromBSHour_hr : BusSelector  OutputSignals=VHAL_TimeSyncFromBSHour_hr
  slr_VHAL_TimeSyncFromBSMinute_min : BusSelector  OutputSignals=VHAL_TimeSyncFromBSMinute_min
  slr_VHAL_TimeSyncFromBSMonth_MONTH : BusSelector  OutputSignals=VHAL_TimeSyncFromBSMonth_MONTH
  slr_VHAL_TimeSyncFromBSSecond_s : BusSelector  OutputSignals=VHAL_TimeSyncFromBSSecond_s
  slr_VHAL_TimeSyncFromBSYear_YEAR : BusSelector  OutputSignals=VHAL_TimeSyncFromBSYear_YEAR
  VINP_TimeSyncFromBSDay_DAY : Outport
  VINP_TimeSyncFromBSHour_hr : Outport  Port=2
  VINP_TimeSyncFromBSMinute_min : Outport  Port=3
  VINP_TimeSyncFromBSMonth_MONTH : Outport  Port=4
  VINP_TimeSyncFromBSSecond_s : Outport  Port=5
  VINP_TimeSyncFromBSYear_YEAR : Outport  Port=6
  wires:
  BHAL_outputs/1 -> [BHAL_outputs]
  inp_CanValid_bus/1 -> [inp_CanValid_bus]
  [BHAL_outputs] -> slr_VHAL_TimeSyncFromBSDay_DAY/1
  slr_VHAL_TimeSyncFromBSDay_DAY/1 -> TimeSyncFromBSDay/1  "<VHAL_TimeSyncFromBSDay_DAY>"
  True_VHAL_TimeSyncFromBSDay_DAY/1 -> TimeSyncFromBSDay/2
  [inp_CanValid_bus] -> slr1_1/1
  slr1_1/1 -> TimeSyncFromBSDay/3  "<VINP_CANMsgValidTBOX2_flg>"
  TimeSyncFromBSDay/1 -> VINP_TimeSyncFromBSDay_DAY/1  "VINP_TimeSyncFromBSDay_DAY"
  TimeSyncFromBSDay/2 -> Terminator_1/1
  [BHAL_outputs] -> slr_VHAL_TimeSyncFromBSHour_hr/1
  slr_VHAL_TimeSyncFromBSHour_hr/1 -> TimeSyncFromBSHour/1  "<VHAL_TimeSyncFromBSHour_hr>"
  True_VHAL_TimeSyncFromBSHour_hr/1 -> TimeSyncFromBSHour/2
  [inp_CanValid_bus] -> slr1_2/1
  slr1_2/1 -> TimeSyncFromBSHour/3  "<VINP_CANMsgValidTBOX2_flg>"
  TimeSyncFromBSHour/1 -> VINP_TimeSyncFromBSHour_hr/1  "VINP_TimeSyncFromBSHour_hr"
  TimeSyncFromBSHour/2 -> Terminator_2/1
  [BHAL_outputs] -> slr_VHAL_TimeSyncFromBSMinute_min/1
  slr_VHAL_TimeSyncFromBSMinute_min/1 -> TimeSyncFromBSMinute/1  "<VHAL_TimeSyncFromBSMinute_min>"
  True_VHAL_TimeSyncFromBSMinute_min/1 -> TimeSyncFromBSMinute/2
  [inp_CanValid_bus] -> slr1_3/1
  slr1_3/1 -> TimeSyncFromBSMinute/3  "<VINP_CANMsgValidTBOX2_flg>"
  TimeSyncFromBSMinute/1 -> VINP_TimeSyncFromBSMinute_min/1  "VINP_TimeSyncFromBSMinute_min"
  TimeSyncFromBSMinute/2 -> Terminator_3/1
  [BHAL_outputs] -> slr_VHAL_TimeSyncFromBSMonth_MONTH/1
  slr_VHAL_TimeSyncFromBSMonth_MONTH/1 -> TimeSyncFromBSMonth/1  "<VHAL_TimeSyncFromBSMonth_MONTH>"
  True_VHAL_TimeSyncFromBSMonth_MONTH/1 -> TimeSyncFromBSMonth/2
  [inp_CanValid_bus] -> slr1_4/1
  slr1_4/1 -> TimeSyncFromBSMonth/3  "<VINP_CANMsgValidTBOX2_flg>"
  TimeSyncFromBSMonth/1 -> VINP_TimeSyncFromBSMonth_MONTH/1  "VINP_TimeSyncFromBSMonth_MONTH"
  TimeSyncFromBSMonth/2 -> Terminator_4/1
  [BHAL_outputs] -> slr_VHAL_TimeSyncFromBSSecond_s/1
  slr_VHAL_TimeSyncFromBSSecond_s/1 -> TimeSyncFromBSSecond/1  "<VHAL_TimeSyncFromBSSecond_s>"
  True_VHAL_TimeSyncFromBSSecond_s/1 -> TimeSyncFromBSSecond/2
  [inp_CanValid_bus] -> slr1_5/1
  slr1_5/1 -> TimeSyncFromBSSecond/3  "<VINP_CANMsgValidTBOX2_flg>"
  TimeSyncFromBSSecond/1 -> VINP_TimeSyncFromBSSecond_s/1  "VINP_TimeSyncFromBSSecond_s"
  TimeSyncFromBSSecond/2 -> Terminator_5/1
  [BHAL_outputs] -> slr_VHAL_TimeSyncFromBSYear_YEAR/1
  slr_VHAL_TimeSyncFromBSYear_YEAR/1 -> TimeSyncFromBSYear/1  "<VHAL_TimeSyncFromBSYear_YEAR>"
  True_VHAL_TimeSyncFromBSYear_YEAR/1 -> TimeSyncFromBSYear/2
  [inp_CanValid_bus] -> slr1_6/1
  slr1_6/1 -> TimeSyncFromBSYear/3  "<VINP_CANMsgValidTBOX2_flg>"
  TimeSyncFromBSYear/1 -> VINP_TimeSyncFromBSYear_YEAR/1  "VINP_TimeSyncFromBSYear_YEAR"
  TimeSyncFromBSYear/2 -> Terminator_6/1
